simulink subsystem "PvtSubSys_VSM_ALL"  (R2020b)
settings: Solver=VariableStepAuto  StartTime=0.0  StopTime=10.0  RelTol=1e-3
values from neighbouring files (symbols this model uses):
  P_VSM_NOH_Act_Req = 0    [VSM_All.sldd]
  P_VSM_NOH_Swt_Req = 0    [VSM_All.sldd]
undefined symbols (not defined in the file or in its folder): ACC_STATE, HWA_STATE, LCK_STATE, P_VSM_ACCSOS_SW, P_VSM_AESSwtReq, P_VSM_CruiseFunUserInputMappingWays, P_VSM_ELKSwtReq, P_VSM_ESS_VehSwtReq, P_VSM_HWA_DMS_Enable, P_VSM_ICA_HandsOffSwtReq, P_VSM_IntelligentEvaSwtReq, P_VSM_ISLSwtReq, P_VSM_LCKSwtReq, P_VSM_LDWSwtReq, P_VSM_LKASwtReq, P_VSM_LSSSwtReq, P_VSM_PowerTrainConfig, P_VSM_SOSContinueTime, P_VSM_SOSSpdLimit, P_VSM_TSR_Dis_keep_SPL_Table, P_VSM_TSR_Dis_keep_SPLend, P_VSM_TSR_Dis_keep_TS_Table, P_VSM_TSR_Ena_SPLSupp_Table, P_VSM_TSR_Ena_TS_Table, P_VSM_TSR_SLIF_Speed_High, P_VSM_TSR_SLIF_Speed_Low, P_VSM_TSR_SLW_SnvtySwitch, P_VSM_TSR_SLW_Speed_Delta_disable, P_VSM_TSR_SLW_Speed_Delta_enable, P_VSM_TSR_SLW_Speed_High, P_VSM_TSR_SLW_Speed_Low, P_VSM_TSR_SLW_TrafEyeAvtiveDist, P_VSM_TSR_SLW_Warning_Time, P_VSM_TSR_SteerWheelAngle, P_VSM_TSR_SWS_speed_withDir, P_VSM_TSR_SWS_speed_woDir, P_VSM_TSRSwtReq, P_VSM_TSRWarnSwtReq, TJA_STATE, User_LC_ALCswt, User_LC_DrvConfirm, User_LC_DrvLCswt, User_LC_DrvOverride, User_LC_LeTurnNextLineReq, User_LC_RiTurnNextLineReq, User_LC_TurnMostLeLineReq, User_LC_TurnMostRiLineReq, User_LeTurnLmpOn, User_RiTurnLmpOn
libraries: simulink x51
(part 1 of 7)
settings Model: Creator=GW00184765  LastModifiedBy=GW00201118

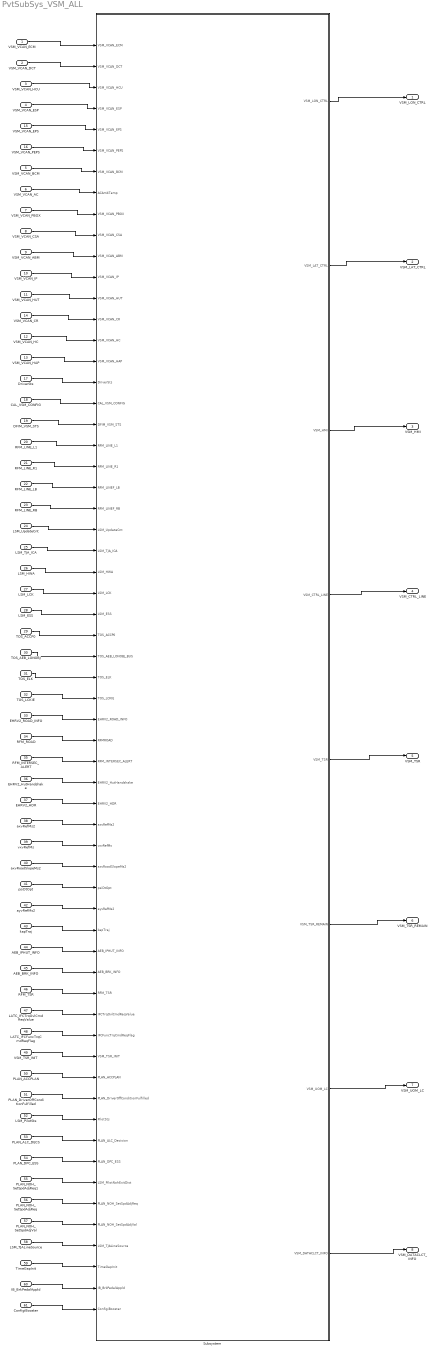
== system PvtSubSys_VSM_ALL ==
  VSM_VCAN_ECM : Inport  OutDataTypeStr=Bus: VCAN_ECM_MSG_BUS  PortDimensions=1  BusOutputAsStruct=on
  VSM_VCAN_DCT : Inport  Port=2  OutDataTypeStr=Bus: VCAN_DCT_MSG_BUS  PortDimensions=1  BusOutputAsStruct=on
  VSM_VCAN_HCU : Inport  Port=3  OutDataTypeStr=Bus: VCAN_HCU_MSG_BUS  PortDimensions=1  BusOutputAsStruct=on
  VSM_VCAN_ESP : Inport  Port=4  OutDataTypeStr=Bus: VCAN_ESP_MSG_BUS  PortDimensions=1  BusOutputAsStruct=on
  VSM_VCAN_BCM : Inport  Port=5  OutDataTypeStr=Bus: VCAN_BCM_MSG_BUS  PortDimensions=1  BusOutputAsStruct=on
  VSM_VCAN_AC : Inport  Port=6  OutDataTypeStr=Bus: VCAN_AC_MSG_BUS  PortDimensions=1  BusOutputAsStruct=on
  VSM_VCAN_PBOX : Inport  Port=7  OutDataTypeStr=Bus: VCAN_PBOX_MSG_BUS  PortDimensions=1  BusOutputAsStruct=on
  VSM_VCAN_CSA : Inport  Port=8  OutDataTypeStr=Bus: VCAN_CSA_MSG_BUS  PortDimensions=1  BusOutputAsStruct=on
  VSM_VCAN_ABM : Inport  Port=9  OutDataTypeStr=Bus: VCAN_ABM_MSG_BUS  PortDimensions=1  BusOutputAsStruct=on
  VSM_VCAN_IP : Inport  Port=10  OutDataTypeStr=Bus: VCAN_IP_MSG_BUS  PortDimensions=1  BusOutputAsStruct=on
  VSM_VCAN_HUT : Inport  Port=11  OutDataTypeStr=Bus: VCAN_HUT_MSG_BUS  PortDimensions=1  BusOutputAsStruct=on
  VSM_VCAN_HC : Inport  Port=12  OutDataTypeStr=Bus: VCAN_HC_MSG_BUS  PortDimensions=1  BusOutputAsStruct=on
  VSM_VCAN_HAP : Inport  Port=13  OutDataTypeStr=Bus: VCAN_HAP_MSG_BUS  PortDimensions=1  BusOutputAsStruct=on
  VSM_VCAN_CR : Inport  Port=14  OutDataTypeStr=Bus: VCAN_CR_MSG_BUS  PortDimensions=1  BusOutputAsStruct=on
  VSM_VCAN_EPS : Inport  Port=15  OutDataTypeStr=Bus: VCAN_EPS_MSG_BUS  PortDimensions=1  BusOutputAsStruct=on
  VSM_VCAN_PEPS : Inport  Port=16  OutDataTypeStr=Bus: VCAN_PEPS_MSG_BUS  PortDimensions=1  BusOutputAsStruct=on
  DriverSts : Inport  Port=17  OutDataTypeStr=uint8  PortDimensions=1  BusOutputAsStruct=on
  CAL_VSM_CONFIG : Inport  Port=18  OutDataTypeStr=Bus: CAL_VSM_CONFIG_BUS  PortDimensions=1  BusOutputAsStruct=on
  DFIM_VSM_STS : Inport  Port=19  OutDataTypeStr=Bus: DFIM_VSM_STS_BUS  PortDimensions=1  BusOutputAsStruct=on
  RFM_LINE_L1 : Inport  Port=20  OutDataTypeStr=Bus: RFM_LINE_BUS  PortDimensions=1  BusOutputAsStruct=on
  RFM_LINE_R1 : Inport  Port=21  OutDataTypeStr=Bus: RFM_LINE_BUS  PortDimensions=1  BusOutputAsStruct=on
  RFM_LINE_LB : Inport  Port=22  OutDataTypeStr=Bus: RFM_LINE_BUS  PortDimensions=1  BusOutputAsStruct=on
  RFM_LINE_RB : Inport  Port=23  OutDataTypeStr=Bus: RFM_LINE_BUS  PortDimensions=1  BusOutputAsStruct=on
  LSM_UpdateCnt : Inport  Port=24  OutDataTypeStr=uint32  PortDimensions=1  BusOutputAsStruct=on
  LSM_TJA_ICA : Inport  Port=25  OutDataTypeStr=Bus: LSM_TJA_ICA_BUS  PortDimensions=1  BusOutputAsStruct=on
  LSM_HWA : Inport  Port=26  OutDataTypeStr=Bus: LSM_HWA_BUS  PortDimensions=1  BusOutputAsStruct=on
  LSM_LCK : Inport  Port=27  OutDataTypeStr=Bus: LSM_LCK_BUS  PortDimensions=1  BusOutputAsStruct=on
  LSM_ESS : Inport  Port=28  OutDataTypeStr=Bus: LSM_ESS_BUS  PortDimensions=1  BusOutputAsStruct=on
  TOS_ACCP0 : Inport  Port=29  OutDataTypeStr=Bus: TOS_ACCP0_BUS  PortDimensions=1  BusOutputAsStruct=on
  TOS_AEB_LONOBJ : Inport  Port=30  OutDataTypeStr=Bus: TOS_AEB_LONOBJ_BUS  PortDimensions=1  BusOutputAsStruct=on
  TOS_ELK : Inport  Port=31  OutDataTypeStr=Bus: TOS_ELK_BUS  PortDimensions=1  BusOutputAsStruct=on
  TOS_LCKIE : Inport  Port=32  OutDataTypeStr=Bus: TOS_LCKIE_BUS  PortDimensions=1  BusOutputAsStruct=on
  EHRV2_ROAD_INFO : Inport  Port=33  OutDataTypeStr=Bus: EHRV2_ROAD_INFO_BUS  PortDimensions=1  BusOutputAsStruct=on
  RFM_ROAD : Inport  Port=34  OutDataTypeStr=Bus: RFM_ROAD_BUS  PortDimensions=1  BusOutputAsStruct=on
  RFM_INTERSEC_ALERT : Inport  Port=35  OutDataTypeStr=Bus: RFM_INTERSEC_ALERT_BUS  PortDimensions=1  BusOutputAsStruct=on
  EHRV2_HutHandshake : Inport  Port=36  OutDataTypeStr=uint8  PortDimensions=1  BusOutputAsStruct=on
  EHRV2_HDR : Inport  Port=37  OutDataTypeStr=Bus: EHRV2_HDR_BUS  PortDimensions=1  BusOutputAsStruct=on
  axvRefMs2 : Inport  Port=38  OutDataTypeStr=single  PortDimensions=1  BusOutputAsStruct=on
  vxvRefMs : Inport  Port=39  OutDataTypeStr=single  PortDimensions=1  BusOutputAsStruct=on
  axvRoadSlopeMs2 : Inport  Port=40  OutDataTypeStr=single  PortDimensions=1  BusOutputAsStruct=on
  psiDtOpt : Inport  Port=41  OutDataTypeStr=single  PortDimensions=1  BusOutputAsStruct=on
  ayvRefMs2 : Inport  Port=42  OutDataTypeStr=single  PortDimensions=1  BusOutputAsStruct=on
  kapTraj : Inport  Port=43  OutDataTypeStr=single  PortDimensions=1  BusOutputAsStruct=on
  AEB_IPHUT_INFO : Inport  Port=44  OutDataTypeStr=Bus: AEB_IPHUT_INFO_BUS  PortDimensions=1  BusOutputAsStruct=on
  AEB_BRK_INFO : Inport  Port=45  OutDataTypeStr=Bus: AEB_BRK_INFO_BUS  PortDimensions=1  BusOutputAsStruct=on
  RFM_TSR : Inport  Port=46  OutDataTypeStr=Bus: RFM_TSR_BUS  PortDimensions=1  BusOutputAsStruct=on
  LATC_IFCTrqOvlCmdReqValue : Inport  Port=47  OutDataTypeStr=single  PortDimensions=1  BusOutputAsStruct=on
  LATC_IFCFuncTrqCmdReqFlag : Inport  Port=48  OutDataTypeStr=uint8  PortDimensions=1  BusOutputAsStruct=on
  VSM_TSR_INIT : Inport  Port=49  OutDataTypeStr=Bus: VSM_TSR_INIT_BUS  PortDimensions=1  BusOutputAsStruct=on
  PLAN_ACCPLAN : Inport  Port=50  OutDataTypeStr=Bus: PLAN_ACCPLAN_BUS  PortDimensions=1  BusOutputAsStruct=on
  PLAN_DriverOffConditionFulfilled : Inport  Port=51  OutDataTypeStr=boolean  PortDimensions=1  BusOutputAsStruct=on
  LSM_PilotSts : Inport  Port=52  OutDataTypeStr=uint8  PortDimensions=1  BusOutputAsStruct=on
  PLAN_ALC_DECS : Inport  Port=53  OutDataTypeStr=Bus: PLAN_ALC_DECS_BUS  PortDimensions=1  BusOutputAsStruct=on
  PLAN_DPC_ESS : Inport  Port=54  OutDataTypeStr=Bus: PLAN_DPC_ESS_BUS  PortDimensions=1  BusOutputAsStruct=on
  PLAN_NOH_SetSpdAdjReq1 : Inport  Port=55  OutDataTypeStr=uint16
  PLAN_NOH_SetSpdAdjReq : Inport  Port=56  OutDataTypeStr=boolean
  PLAN_NOH_SetSpdAdjVal : Inport  Port=57  OutDataTypeStr=uint8
  LSM_TJALineSource : Inport  Port=58  OutDataTypeStr=uint8
  TimeGapInit : Inport  Port=59
  IB_BrkPedalAppld : Inport  Port=60
  ConfigiBooster : Inport  Port=61
  Subsystem : Subsystem
  VSM_LON_CTRL : Outport  OutDataTypeStr=Bus: VSM_LON_CTRL_BUS  PortDimensions=1  BusOutputAsStruct=on
  VSM_LAT_CTRL : Outport  Port=2  OutDataTypeStr=Bus: VSM_LAT_CTRL_BUS  BusOutputAsStruct=on
  VSM_HMI : Outport  Port=3  OutDataTypeStr=Bus: VSM_HMI_BUS  PortDimensions=1  BusOutputAsStruct=on
  VSM_CTRL_LINE : Outport  Port=4  OutDataTypeStr=Bus: VSM_CTRL_LINE_BUS  PortDimensions=1  BusOutputAsStruct=on
  VSM_TSR : Outport  Port=5  OutDataTypeStr=Bus: VSM_TSR_BUS  PortDimensions=1  BusOutputAsStruct=on
  VSM_TSR_REMAIN : Outport  Port=6  OutDataTypeStr=Bus: VSM_TSR_REMAIN_BUS  BusOutputAsStruct=on
  VSM_UOM_LC : Outport  Port=7  OutDataTypeStr=Bus: VSM_UOM_LC_BUS  PortDimensions=1  BusOutputAsStruct=on
  VSM_DATACLCT_INFO : Outport  Port=8  OutDataTypeStr=Bus: VSM_DATACLCT_INFO_BUS  PortDimensions=1  BusOutputAsStruct=on
  wires:
  Subsystem/1(VSM_LON_CTRL) -> VSM_LON_CTRL/1
  Subsystem/2(VSM_LAT_CTRL) -> VSM_LAT_CTRL/1
  Subsystem/3(VSM_HMI) -> VSM_HMI/1
  Subsystem/4(VSM_CTRL_LINE) -> VSM_CTRL_LINE/1
  Subsystem/5(VSM_TSR) -> VSM_TSR/1
  Subsystem/6(VSM_TSR_REMAIN) -> VSM_TSR_REMAIN/1
  Subsystem/7(VSM_UOM_LC) -> VSM_UOM_LC/1
  Subsystem/8(VSM_DATACLCT_INFO) -> VSM_DATACLCT_INFO/1
  VSM_VCAN_ECM/1 -> Subsystem/1(VSM_VCAN_ECM)
  VSM_VCAN_DCT/1 -> Subsystem/2(VSM_VCAN_DCT)
  VSM_VCAN_HCU/1 -> Subsystem/3(VSM_VCAN_HCU)
  VSM_VCAN_ESP/1 -> Subsystem/4(VSM_VCAN_ESP)
  VSM_VCAN_BCM/1 -> Subsystem/7(VSM_VCAN_BCM)
  VSM_VCAN_AC/1 -> Subsystem/8(ACAmbTemp)
  VSM_VCAN_PBOX/1 -> Subsystem/9(VSM_VCAN_PBOX)
  VSM_VCAN_CSA/1 -> Subsystem/10(VSM_VCAN_CSA)
  VSM_VCAN_EPS/1 -> Subsystem/5(VSM_VCAN_EPS)
  VSM_VCAN_PEPS/1 -> Subsystem/6(VSM_VCAN_PEPS)
  VSM_VCAN_ABM/1 -> Subsystem/11(VSM_VCAN_ABM)
  VSM_VCAN_IP/1 -> Subsystem/12(VSM_VCAN_IP)
  VSM_VCAN_HUT/1 -> Subsystem/13(VSM_VCAN_HUT)
  VSM_VCAN_HC/1 -> Subsystem/15(VSM_VCAN_HC)
  VSM_VCAN_HAP/1 -> Subsystem/16(VSM_VCAN_HAP)
  VSM_VCAN_CR/1 -> Subsystem/14(VSM_VCAN_CR)
  DriverSts/1 -> Subsystem/17(DriverSts)
  CAL_VSM_CONFIG/1 -> Subsystem/18(CAL_VSM_CONFIG)
  DFIM_VSM_STS/1 -> Subsystem/19(DFIM_VSM_STS)
  RFM_LINE_L1/1 -> Subsystem/20(RFM_LINE_L1)
  RFM_LINE_R1/1 -> Subsystem/21(RFM_LINE_R1)
  RFM_LINE_LB/1 -> Subsystem/22(RFM_LINEF_LB)
  RFM_LINE_RB/1 -> Subsystem/23(RFM_LINEF_RB)
  LSM_UpdateCnt/1 -> Subsystem/24(LSM_UpdateCnt)
  LSM_TJA_ICA/1 -> Subsystem/25(LSM_TJA_ICA)
  LSM_HWA/1 -> Subsystem/26(LSM_HWA)
  LSM_LCK/1 -> Subsystem/27(LSM_LCK)
  LSM_ESS/1 -> Subsystem/28(LSM_ESS)
  TOS_ACCP0/1 -> Subsystem/29(TOS_ACCP0)
  TOS_AEB_LONOBJ/1 -> Subsystem/30(TOS_AEB_LONOBJ_BUS)
  TOS_ELK/1 -> Subsystem/31(TOS_ELK)
  TOS_LCKIE/1 -> Subsystem/32(TOS_LCKIE)
  EHRV2_ROAD_INFO/1 -> Subsystem/33(EHRV2_ROAD_INFO)
  RFM_ROAD/1 -> Subsystem/34(RFMROAD)
  RFM_INTERSEC_ALERT/1 -> Subsystem/35(RFM_INTERSEC_ALERT)
  EHRV2_HutHandshake/1 -> Subsystem/36(EHRV2_HutHandshake)
  EHRV2_HDR/1 -> Subsystem/37(EHRV2_HDR)
  axvRefMs2/1 -> Subsystem/38(axvRefMs2)
  vxvRefMs/1 -> Subsystem/39(vxvRefMs)
  axvRoadSlopeMs2/1 -> Subsystem/40(axvRoadSlopeMs2)
  psiDtOpt/1 -> Subsystem/41(psiDtOpt)
  ayvRefMs2/1 -> Subsystem/42(ayvRefMs2)
  kapTraj/1 -> Subsystem/43(kapTraj)
  AEB_IPHUT_INFO/1 -> Subsystem/44(AEB_IPHUT_INFO)
  AEB_BRK_INFO/1 -> Subsystem/45(AEB_BRK_INFO)
  RFM_TSR/1 -> Subsystem/46(RFM_TSR)
  LATC_IFCTrqOvlCmdReqValue/1 -> Subsystem/47(IFCTrqOvlCmdReqValue)
  LATC_IFCFuncTrqCmdReqFlag/1 -> Subsystem/48(IFCFuncTrqCmdReqFlag)
  VSM_TSR_INIT/1 -> Subsystem/49(VSM_TSR_INIT)
  PLAN_ACCPLAN/1 -> Subsystem/50(PLAN_ACCPLAN)
  PLAN_DriverOffConditionFulfilled/1 -> Subsystem/51(PLAN_DriverOffConditionFulfilled)
  LSM_PilotSts/1 -> Subsystem/52(PilotSts)
  PLAN_ALC_DECS/1 -> Subsystem/53(PLAN_ALC_Decision)
  PLAN_DPC_ESS/1 -> Subsystem/54(PLAN_DPC_ESS)
  PLAN_NOH_SetSpdAdjReq/1 -> Subsystem/56(PLAN_NOH_SetSpdAdjReq)
  PLAN_NOH_SetSpdAdjVal/1 -> Subsystem/57(PLAN_NOH_SetSpdAdjVal)
  PLAN_NOH_SetSpdAdjReq1/1 -> Subsystem/55(LSM_PilotNohExitDist)
  LSM_TJALineSource/1 -> Subsystem/58(LSM_TJALineSource)
  TimeGapInit/1 -> Subsystem/59(TimeGapInit)
  IB_BrkPedalAppld/1 -> Subsystem/60(IB_BrkPedalAppld)
  ConfigiBooster/1 -> Subsystem/61(ConfigiBooster)

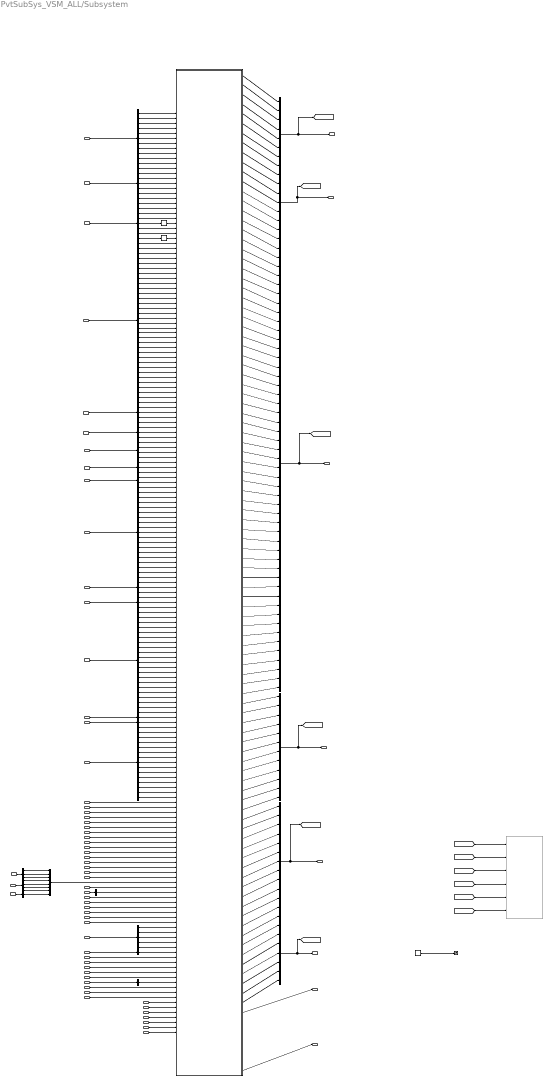
== system PvtSubSys_VSM_ALL/Subsystem ==
  note: 测试版
      | 2021.1.20
      | 1、ACC增加HAP_CAN bus和p0_dx，因此修改框架;
      | 2021.1.22
      | 1、添加LCK居中条件；
      | 2、修改ISL开关逻辑；
      | 2021.1.23
      | UOM添加信号；
      | 2021.1.27
      | TJA_FollowSts修改；
      | 2021.2.1
      | DBC升级4.11
      | 2021.2.22
      | 接口更新NOH；
  VSM_VCAN_ECM : Inport  OutDataTypeStr=Bus: VCAN_ECM_MSG_BUS  BusOutputAsStruct=on
  VSM_VCAN_DCT : Inport  Port=2  OutDataTypeStr=Bus: VCAN_DCT_MSG_BUS  PortDimensions=1  Interpolate=off  BusOutputAsStruct=on
  VSM_VCAN_HCU : Inport  Port=3  OutDataTypeStr=Bus: VCAN_HCU_MSG_BUS  BusOutputAsStruct=on
  VSM_VCAN_ESP : Inport  Port=4  OutDataTypeStr=Bus: VCAN_ESP_MSG_BUS  PortDimensions=1  Interpolate=off  BusOutputAsStruct=on
  VSM_VCAN_EPS : Inport  Port=5  OutDataTypeStr=Bus: VCAN_EPS_MSG_BUS  PortDimensions=1  Interpolate=off  BusOutputAsStruct=on
  VSM_VCAN_PEPS : Inport  Port=6  OutDataTypeStr=Bus: VCAN_PEPS_MSG_BUS  PortDimensions=1  Interpolate=off  BusOutputAsStruct=on
  VSM_VCAN_BCM : Inport  Port=7  OutDataTypeStr=Bus: VCAN_BCM_MSG_BUS  PortDimensions=1  Interpolate=off  BusOutputAsStruct=on
  ACAmbTemp : Inport  Port=8  OutDataTypeStr=Bus: VCAN_AC_MSG_BUS  PortDimensions=1  Interpolate=off  BusOutputAsStruct=on
  VSM_VCAN_PBOX : Inport  Port=9  OutDataTypeStr=Bus: VCAN_PBOX_MSG_BUS  PortDimensions=1  Interpolate=off  BusOutputAsStruct=on
  VSM_VCAN_CSA : Inport  Port=10  OutDataTypeStr=Bus: VCAN_CSA_MSG_BUS  PortDimensions=1  Interpolate=off  BusOutputAsStruct=on
  VSM_VCAN_ABM : Inport  Port=11  OutDataTypeStr=Bus: VCAN_ABM_MSG_BUS  PortDimensions=1  Interpolate=off  BusOutputAsStruct=on
  VSM_VCAN_IP : Inport  Port=12  OutDataTypeStr=Bus: VCAN_IP_MSG_BUS  PortDimensions=1  Interpolate=off  BusOutputAsStruct=on
  VSM_VCAN_HUT : Inport  Port=13  OutDataTypeStr=Bus: VCAN_HUT_MSG_BUS  PortDimensions=1  Interpolate=off  BusOutputAsStruct=on
  VSM_VCAN_CR : Inport  Port=14  OutDataTypeStr=Bus: VCAN_CR_MSG_BUS  PortDimensions=1  Interpolate=off  BusOutputAsStruct=on
  VSM_VCAN_HC : Inport  Port=15  OutDataTypeStr=Bus: VCAN_HC_MSG_BUS  PortDimensions=1  Interpolate=off  BusOutputAsStruct=on
  VSM_VCAN_HAP : Inport  Port=16  OutDataTypeStr=Bus: VCAN_HAP_MSG_BUS  PortDimensions=1  Interpolate=off  BusOutputAsStruct=on
  DriverSts : Inport  Port=17  OutDataTypeStr=uint8  PortDimensions=1  Interpolate=off  BusOutputAsStruct=on
  CAL_VSM_CONFIG : Inport  Port=18  OutDataTypeStr=Bus: CAL_VSM_CONFIG_BUS  PortDimensions=1  Interpolate=off  BusOutputAsStruct=on
  DFIM_VSM_STS : Inport  Port=19  OutDataTypeStr=Bus: DFIM_VSM_STS_BUS  PortDimensions=1  Interpolate=off  BusOutputAsStruct=on
  RFM_LINE_L1 : Inport  Port=20  OutDataTypeStr=Bus: RFM_LINE_BUS  PortDimensions=1  Interpolate=off  BusOutputAsStruct=on
  RFM_LINE_R1 : Inport  Port=21  OutDataTypeStr=Bus: RFM_LINE_BUS  PortDimensions=1  Interpolate=off  BusOutputAsStruct=on
  RFM_LINEF_LB : Inport  Port=22  OutDataTypeStr=Bus: RFM_LINE_BUS  PortDimensions=1  Interpolate=off  BusOutputAsStruct=on
  RFM_LINEF_RB : Inport  Port=23  OutDataTypeStr=Bus: RFM_LINE_BUS  PortDimensions=1  Interpolate=off  BusOutputAsStruct=on
  LSM_UpdateCnt : Inport  Port=24  OutDataTypeStr=uint32  PortDimensions=1  Interpolate=off  BusOutputAsStruct=on
  LSM_TJA_ICA : Inport  Port=25  OutDataTypeStr=Bus: LSM_TJA_ICA_BUS  PortDimensions=1  Interpolate=off  BusOutputAsStruct=on
  LSM_HWA : Inport  Port=26  OutDataTypeStr=Bus: LSM_HWA_BUS  PortDimensions=1  Interpolate=off  BusOutputAsStruct=on
  LSM_LCK : Inport  Port=27  OutDataTypeStr=Bus: LSM_LCK_BUS  PortDimensions=1  Interpolate=off  BusOutputAsStruct=on
  LSM_ESS : Inport  Port=28  OutDataTypeStr=Bus: LSM_ESS_BUS  PortDimensions=1  Interpolate=off  BusOutputAsStruct=on
  TOS_ACCP0 : Inport  Port=29  OutDataTypeStr=Bus: TOS_ACCP0_BUS  PortDimensions=1  BusOutputAsStruct=on
  TOS_AEB_LONOBJ_BUS : Inport  Port=30  OutDataTypeStr=Bus: TOS_AEB_LONOBJ_BUS  PortDimensions=1  BusOutputAsStruct=on
  TOS_ELK : Inport  Port=31  OutDataTypeStr=Bus: TOS_ELK_BUS  PortDimensions=1  BusOutputAsStruct=on
  TOS_LCKIE : Inport  Port=32  OutDataTypeStr=Bus: TOS_LCKIE_BUS  PortDimensions=1  BusOutputAsStruct=on
  EHRV2_ROAD_INFO : Inport  Port=33  OutDataTypeStr=Bus: EHRV2_ROAD_INFO_BUS  PortDimensions=1  Interpolate=off  BusOutputAsStruct=on
  RFMROAD : Inport  Port=34  OutDataTypeStr=Bus: RFM_ROAD_BUS
  RFM_INTERSEC_ALERT : Inport  Port=35  OutDataTypeStr=Bus: RFM_INTERSEC_ALERT_BUS  PortDimensions=1  BusOutputAsStruct=on
  EHRV2_HutHandshake : Inport  Port=36  OutDataTypeStr=uint8  PortDimensions=1  BusOutputAsStruct=on
  EHRV2_HDR : Inport  Port=37  OutDataTypeStr=Bus: EHRV2_HDR_BUS  PortDimensions=1  BusOutputAsStruct=on
  axvRefMs2 : Inport  Port=38  OutDataTypeStr=single  PortDimensions=1  Interpolate=off  BusOutputAsStruct=on
  vxvRefMs : Inport  Port=39  OutDataTypeStr=single  PortDimensions=1  Interpolate=off  BusOutputAsStruct=on
  axvRoadSlopeMs2 : Inport  Port=40  OutDataTypeStr=single  PortDimensions=1  Interpolate=off  BusOutputAsStruct=on
  psiDtOpt : Inport  Port=41  OutDataTypeStr=single  PortDimensions=1  Interpolate=off  BusOutputAsStruct=on
  ayvRefMs2 : Inport  Port=42  OutDataTypeStr=single  PortDimensions=1  Interpolate=off  BusOutputAsStruct=on
  kapTraj : Inport  Port=43  OutDataTypeStr=single  PortDimensions=1  Interpolate=off  BusOutputAsStruct=on
  AEB_IPHUT_INFO : Inport  Port=44  OutDataTypeStr=Bus: AEB_IPHUT_INFO_BUS  PortDimensions=1  Interpolate=off  BusOutputAsStruct=on
  AEB_BRK_INFO : Inport  Port=45  OutDataTypeStr=Bus: AEB_BRK_INFO_BUS  PortDimensions=1  Interpolate=off  BusOutputAsStruct=on
  RFM_TSR : Inport  Port=46  OutDataTypeStr=Bus: RFM_TSR_BUS  PortDimensions=1  Interpolate=off  BusOutputAsStruct=on
  IFCTrqOvlCmdReqValue : Inport  Port=47  OutDataTypeStr=single  PortDimensions=1  Interpolate=off  BusOutputAsStruct=on
  IFCFuncTrqCmdReqFlag : Inport  Port=48  OutDataTypeStr=uint8  PortDimensions=1  Interpolate=off  BusOutputAsStruct=on
  VSM_TSR_INIT : Inport  Port=49  OutDataTypeStr=Bus: VSM_TSR_INIT_BUS  PortDimensions=1  Interpolate=off  BusOutputAsStruct=on
  PLAN_ACCPLAN : Inport  Port=50  OutDataTypeStr=Bus: PLAN_ACCPLAN_BUS  PortDimensions=1  Interpolate=off  BusOutputAsStruct=on
  PLAN_DriverOffConditionFulfilled : Inport  Port=51  OutDataTypeStr=boolean  PortDimensions=1  Interpolate=off  BusOutputAsStruct=on
  PilotSts : Inport  Port=52
  PLAN_ALC_Decision : Inport  Port=53  OutDataTypeStr=Bus: PLAN_ALC_DECS_BUS
  PLAN_DPC_ESS : Inport  Port=54  OutDataTypeStr=Bus: PLAN_DPC_ESS_BUS
  LSM_PilotNohExitDist : Inport  Port=55  OutDataTypeStr=uint16
  PLAN_NOH_SetSpdAdjReq : Inport  Port=56  OutDataTypeStr=boolean
  PLAN_NOH_SetSpdAdjVal : Inport  Port=57  OutDataTypeStr=uint8
  LSM_TJALineSource : Inport  Port=58
  TimeGapInit : Inport  Port=59
  IB_BrkPedalAppld : Inport  Port=60
  ConfigiBooster : Inport  Port=61
  Bus Creator : BusCreator  Inputs=8  OutDataTypeStr=Bus: VSM_LON_CTRL_BUS  NonVirtualBus=on
  Bus Creator1 : BusCreator  Inputs=7  OutDataTypeStr=Bus: VSM_LAT_CTRL_BUS  NonVirtualBus=on
  Bus Creator2 : BusCreator  Inputs=50  OutDataTypeStr=Bus: VSM_HMI_BUS  NonVirtualBus=on
  Bus Creator3 : BusCreator  Inputs=12  OutDataTypeStr=Bus: VSM_CTRL_LINE_BUS  NonVirtualBus=on
  Bus Creator4 : BusCreator  Inputs=13  OutDataTypeStr=Bus: VSM_TSR_BUS  NonVirtualBus=on
  Bus Creator5 : BusCreator  Inputs=7  OutDataTypeStr=Bus: VSM_TSR_REMAIN_BUS  NonVirtualBus=on
  Bus Creator6 : BusCreator  Inputs=8
  Bus Selector : BusSelector  OutputSignals=FrntWshrSwtSts,FrntWiprSwtSts,LTurnLmpSwtSts,RTurnLmpSwtSts,SteerWheelAng,SteerWheelAngSign,SteerWheelSpd,SteerWheelSpdSign,SAS_Sts,ACC_TimeGap_IncSetSwt,ACC_TimeGap_DecSetSwt,CC_ACC_CRUISE_OFFSwt,CC_ACC_CANCEL_OFFSwt,CC_ACC_IncSetSpd_ResuSwt,CC_ACC_DecSetSpd_SetSwt,CC_ACCSwtErr,HWA_OK_OFFSwt
  Bus Selector1 : BusSelector  OutputSignals=HCU_BrkPedalSts,HCU_AccelPedalPosn_Diag,HCU_ACCInterface,HCU_PowertrainSts,ACU_ShiftInProgress,HCU_DrvMod,HCU_PTDrvMod,DrvTrqReqOvld,HCU_GearSts
  Bus Selector10 : BusSelector  OutputSignals=i_func_road_class,i_form_of_way,i_road_curvature_far
  Bus Selector11 : BusSelector  OutputSignals=MapDataValid
  Bus Selector12 : BusSelector  OutputSignals=f_tunnel_distance,b_tunnel,f_bridge_distance,b_bridge
  Bus Selector13 : BusSelector  OutputSignals=f_start_distance
  Bus Selector14 : BusSelector  OutputSignals=EPS_FailSts,EPS_TrqSnsrSts,EPS_SteerMod,EPS_LKATorqOvrlDlvd,EPS_LKATorqOvrlDlvdVld,EPS_LKATrqOvlDlvdSts,EPS_DrvInpTrqVal_HighReslolution
  Bus Selector15 : BusSelector  OutputSignals=SysPowerMod
  Bus Selector16 : BusSelector  OutputSignals=ACAmbTemp
  Bus Selector17 : BusSelector  OutputSignals=IP_VehSpdUnit
  Bus Selector18 : BusSelector  OutputSignals=CR_BrkgReq
  Bus Selector19 : BusSelector  OutputSignals=HighBeamSts_HC
  Bus Selector2 : BusSelector  OutputSignals=CurrentGearValid,SHIFT_IN_PROGRESS,TargetGearValid,TARGET_GEAR,ShiftInPrgValid,CURRENT_GEAR,TGS_LEVER
  Bus Selector26 : BusSelector  OutputSignals=AEB_VehResp,AEB_PedResp,FCW_Warn,AEB_VehTrig,AEB_PedTrig
  Bus Selector27 : BusSelector  OutputSignals=AEB_TgtDecel_Req
  Bus Selector3 : BusSelector  OutputSignals=DrivingModDis,BrkDskOvrheatd,NoBrkForce,VehStandstill,HDCCtrl,CDDActv,CDDAvailable,AVHSts,ESPFuncOffSts,ESPBrkLmpCtrl,ESPFailSts,ESP_MasterCylBrkPressVld,MSRActv,VDCActv,PTCActv,BTCActv,ESP_MasterCylBrkPress,MSRActv_RA,PTCActv_RA,BTCActv_RA,ABSFailSts,EBDFailSts,VehSpd,ABSActv,EPBSts,EPB_SwtPosn,RLWheelDriveDirection,RLWheelSpd,RRWheelDriveDirection,RRWheelSpd
  Bus Selector30 : BusSelector  OutputSignals=EngState_PHEV,EngSpd,EngState,BrkPedalSts,Start_StopSts,AccPedalOverride,AccelPedlPosnDiagc,ECMRespACC,ECMACCInterface,AccelPedalPosn,EngLimpHomeSts
  Bus Selector4 : BusSelector  OutputSignals=ACC_axvCvAim
  Bus Selector5 : BusSelector  OutputSignals=WiprReq_F_PBOX,DrvDoorSts,PassengerDoorSts,WindshldWiprActvSts,HazardLmpSwtSts,KL30BRelaySts
  Bus Selector6 : BusSelector  OutputSignals=HoodSts_F_Pbox,FFogLmpSts_F_Pbox,RFogLmpSts_R_Pbox,LowBeamSts_F_Pbox
  Bus Selector7 : BusSelector  OutputSignals=DrvSBR,PassSBR,VehLgtAccel,VehLatAccel,VehYawRate
  Bus Selector8 : BusSelector  OutputSignals=IFC_SnvtySet,LKASwtReq,LCKSwtReq,ELKSwtReq,ESS_PedSwtReq,ESS_VehSwtReq,LDWSwtReq,TSRSwtReq,TSRWarnSwtReq,ICA_HandsOffSwtReq,ISLSwtReq,TSR_SnvtySet,LSSWarnFormSwtReq,LSSSwtReq,IntelligentEvaSwtReq,AESSwtReq,HWA_SwtReq,HWA_SnvtySet,ALC_SwtReq,NOH_Act_Req,NOH_Swt_Req,NavRoadType
  Bus Selector9 : BusSelector  OutputSignals=USS_FrontSys_Status,USS_FLCNear_Obj_Confidence,USS_FLCNear_Obj_Pos_X,USS_FLCNear_Obj_Pos_Y,USS_FLMNear_Obj_Confidence,USS_FLMNear_Obj_Pos_X,USS_FLMNear_Obj_Pos_Y,USS_FRMNear_Obj_Confidence,USS_FRMNear_Obj_Pos_X,USS_FRMNear_Obj_Pos_Y,USS_FRCNear_Obj_Confidence,USS_FRCNear_Obj_Pos_X,USS_FRCNear_Obj_Pos_Y,APS_WorkSts,DVRWorkSts
  Compare To Constant : simulink/Logic and Bit Operations/Compare To Constant  relop===  const=1  OutDataTypeStr=boolean
  Compare To Constant1 : simulink/Logic and Bit Operations/Compare To Constant  relop===  const=1  OutDataTypeStr=boolean
  Counter Limited : simulink/Sources/Counter Limited  uplimit=15  tsamp=-1
  StateManage : Subsystem
  Terminator1 : Terminator
  VSM_Signal : Subsystem  Commented=on
  VSM_LON_CTRL : Outport  OutDataTypeStr=Bus: VSM_LON_CTRL_BUS  PortDimensions=1  BusOutputAsStruct=on
  VSM_LAT_CTRL : Outport  Port=2  OutDataTypeStr=Bus: VSM_LAT_CTRL_BUS  BusOutputAsStruct=on
  VSM_HMI : Outport  Port=3  OutDataTypeStr=Bus: VSM_HMI_BUS  PortDimensions=1  BusOutputAsStruct=on
  VSM_CTRL_LINE : Outport  Port=4  OutDataTypeStr=Bus: VSM_CTRL_LINE_BUS  PortDimensions=1  BusOutputAsStruct=on
  VSM_TSR : Outport  Port=5  OutDataTypeStr=Bus: VSM_TSR_BUS  PortDimensions=1  BusOutputAsStruct=on
  VSM_TSR_REMAIN : Outport  Port=6  OutDataTypeStr=Bus: VSM_TSR_REMAIN_BUS  BusOutputAsStruct=on
  VSM_UOM_LC : Outport  Port=7  OutDataTypeStr=Bus: VSM_UOM_LC_BUS
  VSM_DATACLCT_INFO : Outport  Port=8  OutDataTypeStr=Bus: VSM_DATACLCT_INFO_BUS  PortDimensions=1  BusOutputAsStruct=on
  wires:
  Bus Selector10/3 -> Bus Creator6/3  "<i_road_curvature_far>"
  ConfigiBooster/1 -> StateManage/185(ConfigiBooster)
  IB_BrkPedalAppld/1 -> StateManage/184(IB_BrkPedalAppld)
  TimeGapInit/1 -> StateManage/183(TimeGapInit)
  StateManage/8(ACC_TimeGapSetHMI) -> Bus Creator/8
  LSM_TJALineSource/1 -> StateManage/182(LSM_TJALineSource)
  StateManage/65(HWA_LaneChange) -> Bus Creator2/50
  StateManage/58(Signal_DriverOffDisp) -> Bus Creator2/43
  StateManage/64(HiPilotModeSelect) -> Bus Creator2/49
  StateManage/63(NOH_DistToExit) -> Bus Creator2/48
  StateManage/62(NOH_SysInfoDisplay) -> Bus Creator2/47
  StateManage/61(NOH_Act_Resp) -> Bus Creator2/46
  StateManage/60(NOH_Swt_Resp) -> Bus Creator2/45
  StateManage/59(NOH_Sts) -> Bus Creator2/44
  LSM_PilotNohExitDist/1 -> StateManage/179(LSM_PilotNohExitDist)
  Bus Selector8/22 -> StateManage/121(NavRoadType)  "<NavRoadType>"
  Bus Selector8/21 -> StateManage/120(NOH_Swt_Req)  "<NOH_Swt_Req>"
  Bus Selector8/20 -> StateManage/119(NOH_Act_Req)  "<NOH_Act_Req>"
  StateManage/104(VSM_DATACLCT_INFO) -> VSM_DATACLCT_INFO/1
  Compare To Constant1/1 -> StateManage/26(DrvTrqReqOvld)
  Compare To Constant/1 -> StateManage/23(ACU_ShiftInProgress)
  Bus Selector19/1 -> StateManage/123(HighBeamSts)  "<HighBeamSts_HC>"
  VSM_VCAN_CR/1 -> Bus Selector18/1
  VSM_VCAN_IP/1 -> Bus Selector17/1
  ACAmbTemp/1 -> Bus Selector16/1
  VSM_VCAN_PEPS/1 -> Bus Selector15/1
  VSM_VCAN_EPS/1 -> Bus Selector14/1
  PLAN_NOH_SetSpdAdjVal/1 -> StateManage/181(PLAN_NOH_SetSpdAdjVal)
  PLAN_NOH_SetSpdAdjReq/1 -> StateManage/180(PLAN_NOH_SetSpdAdjReq)
  StateManage/98(VSM_UOM_LC) -> VSM_UOM_LC/1
  StateManage/57(HWA_TurnLightReq) -> Bus Creator2/42
  Bus Selector13/1 -> Bus Creator6/8  "<f_start_distance>"
  Bus Selector12/4 -> Bus Creator6/7  "<b_bridge>"
  Bus Selector12/3 -> Bus Creator6/6  "<f_bridge_distance>"
  Bus Selector12/2 -> Bus Creator6/5  "<b_tunnel>"
  Bus Selector12/1 -> Bus Creator6/4  "<f_tunnel_distance>"
  Bus Selector10/2 -> Bus Creator6/2  "<i_form_of_way>"
  Bus Selector10/1 -> Bus Creator6/1  "<i_func_road_class>"
  RFM_INTERSEC_ALERT/1 -> Bus Selector13/1
  RFMROAD/1 -> Bus Selector12/1
  EHRV2_ROAD_INFO/1 -> Bus Selector10/1
  EHRV2_HDR/1 -> Bus Selector11/1
  LSM_TJA_ICA/1 -> StateManage/147(LSM_TJA_ICA)
  [VSM_HMI] -> VSM_Signal/3(VSM_HMI)  "VSM_HMI"
  Bus Selector3/28 -> StateManage/55(RLWheelSpd)  "<RLWheelSpd>"
  Bus Selector18/1 -> StateManage/122(CR_BrkgReq)  "<CR_BrkgReq>"
  Bus Selector30/10 -> StateManage/10(AccelPedalPosn)  "<AccelPedalPosn>"
  StateManage/4(ACC_TimeGapSet) -> Bus Creator/4
  axvRefMs2/1 -> StateManage/158(axvRefMs2)
  StateManage/93(TS_SignName_Dist_Remain) -> Bus Creator5/3
  Bus Selector1/6 -> StateManage/24(HCU_DrvMod)  "<HCU_DrvMod>"
  Bus Selector15/1 -> StateManage/65(SysPowerMod)  "<SysPowerMod>"
  Bus Selector9/10 -> StateManage/133(USS_FRMNear_Obj_Pos_Y)  "<USS_FRMNear_Obj_Pos_Y>"
  Bus Selector1/7 -> StateManage/25(HCU_PTDrvMod)  "<HCU_PTDrvMod>"
  StateManage/42(HWA_SnvtySet_Resp) -> Bus Creator2/27
  StateManage/96(TS_SignName_Value_Remain) -> Bus Creator5/6
  StateManage/92(SPL_whSupp_Dist_Remain) -> Bus Creator5/2
  StateManage/88(TSRConSpdLimWarn) -> Bus Creator4/11
  StateManage/79(TSRResp) -> Bus Creator4/2
  StateManage/82(TSRSpdLimUnit) -> Bus Creator4/5
  VSM_VCAN_ABM/1 -> Bus Selector7/1
  Bus Selector5/5 -> StateManage/70(HazardLmpSwtSts)  "<HazardLmpSwtSts>"
  VSM_VCAN_HCU/1 -> Bus Selector1/1
  Bus Selector5/4 -> StateManage/69(WindshldWiprActvSts)  "<WindshldWiprActvSts>"
  StateManage/3(SetSpeedKmh) -> Bus Creator/3
  Bus Selector3/27 -> StateManage/54(RLWheelDriveDirection)  "<RLWheelDriveDirection>"
  axvRoadSlopeMs2/1 -> StateManage/160(axvRoadSlopeMs2)
  Bus Selector26/3 -> StateManage/166(Inter_FCW_Warn)  "<FCW_Warn>"
  StateManage/81(TSR_Snvty) -> Bus Creator4/4
  StateManage/84(TSRSpdLim) -> Bus Creator4/7
  TOS_ACCP0/1 -> StateManage/151(TOS_ACCP0)
  StateManage/83(TSRSpdLimSts) -> Bus Creator4/6
  StateManage/76(ELKLineC0) -> Bus Creator3/11
  Bus Creator/1 -> [VSM_LON_CTRL], VSM_LON_CTRL/1
  StateManage/44(ICA_HandsOffSwtResp) -> Bus Creator2/29
  vxvRefMs/1 -> StateManage/159(vxvRefMs)
  StateManage/30(LCKSts) -> Bus Creator2/15
  Bus Selector14/5 -> StateManage/62(EPS_LKATorqOvrlDlvdVld)  "<EPS_LKATorqOvrlDlvdVld>"
  Bus Selector/14 -> StateManage/90(CC_ACC_IncSetSpd_ResuSwt)  "<CC_ACC_IncSetSpd_ResuSwt>"
  StateManage/75(ELKLineC1) -> Bus Creator3/10
  StateManage/40(EPBTakeOver_Req) -> Bus Creator2/25
  PLAN_DriverOffConditionFulfilled/1 -> StateManage/170(DriveOffConditionFulfilled)
  VSM_VCAN_ESP/1 -> Bus Selector3/1
  Bus Selector7/3 -> StateManage/96(VehLgtAccel)  "<VehLgtAccel>"
  StateManage/50(DriverInloop_Monitor) -> Bus Creator2/35
  StateManage/67(LKALineC3) -> Bus Creator3/2
  PLAN_ALC_Decision/1 -> StateManage/176(ALC)
  Bus Selector3/24 -> StateManage/51(ABSActv)  "<ABSActv>"
  Bus Selector/16 -> StateManage/92(CC_ACCSwtErr)  "<CC_ACCSwtErr>"
  Bus Selector8/7 -> StateManage/106(LDWSwtReq)  "<LDWSwtReq>"
  StateManage/54(ESSSts) -> Bus Creator2/39
  VSM_VCAN_BCM/1 -> Bus Selector5/1
  kapTraj/1 -> StateManage/163(kapTraj)
  StateManage/70(LKALineC0) -> Bus Creator3/5
  StateManage/38(ISL_InterSysInfoDisp) -> Bus Creator2/23
  Bus Selector8/1 -> StateManage/100(IFC_SnvtySet)  "<IFC_SnvtySet>"
  StateManage/73(ELKLineC3) -> Bus Creator3/8
  Bus Selector3/8 -> StateManage/35(AVHSts)  "<AVHSts>"
  TOS_LCKIE/1 -> StateManage/154(TOS_LCKIE)
  StateManage/1(ACCSts) -> Bus Creator/1
  StateManage/53(TJA_FollowSts) -> Bus Creator2/38
  VSM_VCAN_DCT/1 -> Bus Selector2/1
  StateManage/31(HandsOffWarningLevel) -> Bus Creator2/16
  Bus Selector9/9 -> StateManage/132(USS_FRMNear_Obj_Pos_X)  "<USS_FRMNear_Obj_Pos_X>"
  Bus Selector3/15 -> StateManage/42(PTCActv)  "<PTCActv>"
  StateManage/78(TSRSts) -> Bus Creator4/1
  RFM_LINE_R1/1 -> StateManage/143(RFM_LINE_R1)
  StateManage/55(AESSts) -> Bus Creator2/40
  RFM_TSR/1 -> StateManage/171(RFM_TSR)
  Bus Selector30/1 -> StateManage/1(EngState_PHEV)  "<EngState_PHEV>"
  Bus Selector8/16 -> StateManage/115(AESSwtReq)  "<AESSwtReq>"
  StateManage/69(LKALineC1) -> Bus Creator3/4
  Bus Selector14/4 -> StateManage/61(EPS_LKATorqOvrlDlvd)  "<EPS_LKATorqOvrlDlvd>"
  VSM_VCAN_HAP/1 -> Bus Selector9/1
  StateManage/33(LKASts) -> Bus Creator2/18
  StateManage/52(LaneAvailability) -> Bus Creator2/37
  Bus Selector9/3 -> StateManage/126(USS_FLCNear_Obj_Pos_X)  "<USS_FLCNear_Obj_Pos_X>"
  Bus Selector/12 -> StateManage/88(CC_ACC_CRUISE_OFFSwt)  "<CC_ACC_CRUISE_OFFSwt>"
  StateManage/77(ELKLineRange) -> Bus Creator3/12
  Bus Selector1/3 -> StateManage/21(HCU_ACCInterface)  "<HCU_ACCInterface>"
  LSM_LCK/1 -> StateManage/149(LSM_LCK)
  Bus Selector2/7 -> StateManage/18(TGS_LEVER)  "<TGS_LEVER>"
  Bus Selector2/5 -> StateManage/16(ShiftInPrgValid)  "<ShiftInPrgValid>"
  Bus Selector1/4 -> StateManage/22(HCU_PowertrainSts)  "<HCU_PowertrainSts>"
  Bus Selector1/9 -> StateManage/27(HCU_GearSts)  "<HCU_GearSts>"
  Bus Selector3/14 -> StateManage/41(VDCActv)  "<VDCActv>"
  Bus Selector3/4 -> StateManage/31(VehStandstill)  "<VehStandstill>"
  Bus Selector2/3 -> StateManage/14(TargetGearValid)  "<TargetGearValid>"
  Bus Selector3/26 -> StateManage/53(EPB_SwtPosn)  "<EPB_SwtPosn>"
  StateManage/35(ELKSts) -> Bus Creator2/20
  Bus Selector/17 -> StateManage/93(HWA_OK_OFFSwt)  "<HWA_OK_OFFSwt>"
  StateManage/71(LKALineRange) -> Bus Creator3/6
  Bus Selector8/9 -> StateManage/108(TSRWarnSwtReq)  "<TSRWarnSwtReq>"
  Bus Selector30/8 -> StateManage/8(ECMRespACC)  "<ECMRespACC>"
  TOS_ELK/1 -> StateManage/153(TOS_ELK)
  StateManage/87(TSRConSpdLim) -> Bus Creator4/10
  Bus Selector3/16 -> StateManage/43(BTCActv)  "<BTCActv>"
  Bus Selector8/15 -> StateManage/114(IntelligentEvaSwtReq)  "<IntelligentEvaSwtReq>"
  Bus Selector/6 -> StateManage/82(SteerWheelAngSign)  "<SteerWheelAngSign>"
  CAL_VSM_CONFIG/1 -> StateManage/140(CAL_VSM_CONFIG)
  Bus Selector8/13 -> StateManage/112(LSSWarnFormSwtReq)  "<LSSWarnFormSwtReq>"
  Bus Selector3/12 -> StateManage/39(ESP_MasterCylBrkPressVld)  "<ESP_MasterCylBrkPressVld>"
  Bus Selector/15 -> StateManage/91(CC_ACC_DecSetSpd_SetSwt)  "<CC_ACC_DecSetSpd_SetSwt>"
  Bus Selector8/19 -> StateManage/118(ALC_SwtReq)  "<ALC_SwtReq>"
  Bus Selector9/6 -> StateManage/129(USS_FLMNear_Obj_Pos_X)  "<USS_FLMNear_Obj_Pos_X>"
  Bus Selector/7 -> StateManage/83(SteerWheelSpd)  "<SteerWheelSpd>"
  VSM_VCAN_ECM/1 -> Bus Selector30/1
  Bus Selector2/4 -> StateManage/15(TARGET_GEAR)  "<TARGET_GEAR>"
  StateManage/16(TJASts) -> Bus Creator2/1
  Bus Selector26/5 -> StateManage/168(AEB_PedTrig)  "<AEB_PedTrig>"
  StateManage/18(HWAActive) -> Bus Creator2/3
  Bus Selector2/6 -> StateManage/17(CURRENT_GEAR)  "<CURRENT_GEAR>"
  StateManage/28(CCTextDisp) -> Bus Creator2/13
  AEB_IPHUT_INFO/1 -> Bus Selector26/1
  StateManage/2(ACC_SpdSetValue) -> Bus Creator/2
  Bus Selector8/2 -> StateManage/101(LKASwtReq)  "<LKASwtReq>"
  StateManage/27(TJATextDisp) -> Bus Creator2/12
  StateManage/29(HWATextDisp) -> Bus Creator2/14
  StateManage/36(LCKIEDist) -> Bus Creator2/21
  Bus Selector9/15 -> StateManage/138(DVRWorkSts)  "<DVRWorkSts>"
  Bus Selector/9 -> StateManage/85(SAS_Sts)  "<SAS_Sts>"
  AEB_BRK_INFO/1 -> Bus Selector27/1
  Bus Selector27/1 -> StateManage/169(" ")  "<AEB_TgtDecel_Req>"
  Bus Selector8/4 -> StateManage/103(ELKSwtReq)  "<ELKSwtReq>"
  Bus Selector/3 -> StateManage/79(LTurnLmpSwtSts)  "<LTurnLmpSwtSts>"
  Bus Selector/2 -> StateManage/78(FrntWiprSwtSts)  "<FrntWiprSwtSts>"
  StateManage/23(HWA_ModeDisp) -> Bus Creator2/8
  IFCTrqOvlCmdReqValue/1 -> StateManage/172(epsTrqReqValue)
  [VSM_LAT_CTRL] -> VSM_Signal/2(VSM_LAT_CTRL)  "VSM_LAT_CTRL"
  RFM_LINEF_RB/1 -> StateManage/145(RFM_LINEF_RB)
  StateManage/91(SPL_noSupp_Dist_Remain) -> Bus Creator5/1
  PLAN_DPC_ESS/1 -> StateManage/177(PLAN_DPC_ESS)
  Bus Selector6/1 -> StateManage/73(HoodSts_F_Pbox)  "<HoodSts_F_Pbox>"
  Bus Selector3/13 -> StateManage/40(MSRActv)  "<MSRActv>"
  StateManage/20(ACC_ModeDisp) -> Bus Creator2/5
  VSM_VCAN_HC/1 -> Bus Selector19/1
  Bus Selector14/6 -> StateManage/63(EPS_LKATrqOvlDlvdSts)  "<EPS_LKATrqOvlDlvdSts>"
  Bus Creator1/1 -> [VSM_LAT_CTRL], VSM_LAT_CTRL/1
  Bus Selector14/2 -> StateManage/59(EPS_TrqSnsrSts)  "<EPS_TrqSnsrSts>"
  Bus Creator4/1 -> VSM_TSR/1, [VSM_TSR]
  Bus Selector3/21 -> StateManage/48(ABSFailSts)  "<ABSFailSts>"
  Bus Selector/5 -> StateManage/81(SteerWheelAng)  "<SteerWheelAng>"
  StateManage/95(SPL_whSupp_Value_Remain) -> Bus Creator5/5
  Bus Selector9/12 -> StateManage/135(USS_FRCNear_Obj_Pos_X)  "<USS_FRCNear_Obj_Pos_X>"
  Bus Selector30/9 -> StateManage/9(ECMACCInterface)  "<ECMACCInterface>"
  Bus Selector30/3 -> StateManage/3(EngState)  "<EngState>"
  StateManage/80(TSRWarnResp) -> Bus Creator4/3
  Bus Selector8/12 -> StateManage/111(TSR_SnvtySet)  "<TSR_SnvtySet>"
  Bus Selector3/20 -> StateManage/47(BTCActv_RA)  "<BTCActv_RA>"
  Bus Selector9/1 -> StateManage/124(USS_FrontSys_Status)  "<USS_FrontSys_Status>"
  StateManage/94(SPL_noSupp_Value_Remain) -> Bus Creator5/4
  Bus Creator5/1 -> VSM_TSR_REMAIN/1, [VSM_TSR_REMAIN]
  Bus Selector11/1 -> StateManage/157(MapDataValid)  "<MapDataValid>"
  Bus Selector3/10 -> StateManage/37(ESPBrkLmpCtrl)  "<ESPBrkLmpCtrl>"
  RFM_LINEF_LB/1 -> StateManage/144(RFM_LINEF_LB)
  StateManage/86(TSRSpdLimWarn) -> Bus Creator4/9
  StateManage/72(ELKLineValid) -> Bus Creator3/7
  Bus Selector14/7 -> StateManage/64(EPS_DrvInpTrqVal_HighReslolution)  "<EPS_DrvInpTrqVal_HighReslolution>"
  LSM_UpdateCnt/1 -> StateManage/146(LSM_Cnt)
  Bus Selector8/11 -> StateManage/110(ISLSwtReq)  "<ISLSwtReq>"
  Bus Selector8/8 -> StateManage/107(TSRSwtReq)  "<TSRSwtReq>"
  Bus Creator6/1 -> StateManage/155(EHRV2_ALL)
  StateManage/66(LKALineValid) -> Bus Creator3/1
  StateManage/90(TSRTrfcSignValCfdc) -> Bus Creator4/13
  Bus Selector17/1 -> StateManage/99(IP_VehSpdUnit)  "<IP_VehSpdUnit>"
  Bus Selector30/11 -> StateManage/11(EngLimpHomeSts)  "<EngLimpHomeSts>"
  Bus Selector3/17 -> StateManage/44(ESP_MasterCylBrkPress)  "<ESP_MasterCylBrkPress>"
  StateManage/17(HWASts) -> Bus Creator2/2
  StateManage/32(LDWSts) -> Bus Creator2/17
  Bus Selector3/2 -> StateManage/29(BrkDskOvrheatd)  "<BrkDskOvrheatd>"
  Bus Selector3/11 -> StateManage/38(ESPFailSts)  "<ESPFailSts>"
  Bus Selector9/11 -> StateManage/134(USS_FRCNear_Obj_Confidence)  "<USS_FRCNear_Obj_Confidence>"
  Bus Selector9/2 -> StateManage/125(USS_FLCNear_Obj_Confidence)  "<USS_FLCNear_Obj_Confidence>"
  Bus Selector8/18 -> StateManage/117(HWA_SnvtySet)  "<HWA_SnvtySet>"
  StateManage/12(TarLineC1) -> Bus Creator1/4
  Bus Selector6/2 -> StateManage/74(FFogLmpSts_F_Pbox)  "<FFogLmpSts_F_Pbox>"
  TOS_AEB_LONOBJ_BUS/1 -> StateManage/152(TOS_AEB_LONOBJ_BUS)
  Bus Selector26/1 -> StateManage/164(AEB_VehResp)  "<AEB_VehResp>"
  Bus Selector9/5 -> StateManage/128(USS_FLMNear_Obj_Confidence)  "<USS_FLMNear_Obj_Confidence>"
  VSM_VCAN_PBOX/1 -> Bus Selector6/1
  StateManage/11(TarLineC2) -> Bus Creator1/3
  Bus Selector7/5 -> StateManage/98(VehYawRate)  "<VehYawRate>"
  StateManage/46(HWA_LaneChangeReq) -> Bus Creator2/31
  Bus Selector3/23 -> StateManage/50(VehSpd)  "<VehSpd>"
  StateManage/6(HWAAccControlSts) -> Bus Creator/6
  StateManage/9(TarLineValid) -> Bus Creator1/1
  Bus Selector26/4 -> StateManage/167(AEB_VehTrig)  "<AEB_VehTrig>"
  StateManage/34(LKAWarning) -> Bus Creator2/19
  StateManage/74(ELKLineC2) -> Bus Creator3/9
  Bus Selector5/6 -> StateManage/71("KL30BRelaySts ")  "<KL30BRelaySts>"
  Bus Selector5/3 -> StateManage/68(PassengerDoorSts)  "<PassengerDoorSts>"
  EHRV2_HutHandshake/1 -> StateManage/156(IFCHUTInterface)
  Bus Selector14/1 -> StateManage/58(EPS_FailSts)  "<EPS_FailSts>"
  Bus Selector30/2 -> StateManage/2(EngSpd)  "<EngSpd>"
  [VSM_TSR] -> VSM_Signal/5(VSM_TSR)  "VSM_TSR"
  StateManage/97(SPL_SuppName_Value_Remain) -> Bus Creator5/7
  Bus Selector3/6 -> StateManage/33(CDDActv)  "<CDDActv>"
  Bus Selector6/4 -> StateManage/76(LowBeamSts)  "<LowBeamSts_F_Pbox>"
  StateManage/26(ACCTextDisp) -> Bus Creator2/11
  LSM_ESS/1 -> StateManage/150(LSM_ESS)
  PLAN_ACCPLAN/1 -> Bus Selector4/1
  StateManage/24(HWASlowRetreat_b) -> Bus Creator2/9
  StateManage/21(ACC_ParkShiftReq) -> Bus Creator2/6
  StateManage/43(HWA_Resp) -> Bus Creator2/28
  Bus Selector/10 -> StateManage/86(ACC_TimeGap_IncSetSwt)  "<ACC_TimeGap_IncSetSwt>"
  psiDtOpt/1 -> StateManage/161(psiDtOpt)
  StateManage/49(LSS_WarnFormSwtResp) -> Bus Creator2/34
  Bus Selector/11 -> StateManage/87(ACC_TimeGap_DecSetSwt)  "<ACC_TimeGap_DecSetSwt>"
  Bus Selector3/22 -> StateManage/49(EBDFailSts)  "<EBDFailSts>"
  Bus Selector16/1 -> StateManage/72(ACAmbTemp)  "<ACAmbTemp>"
  Bus Selector3/3 -> StateManage/30(NoBrkForce)  "<NoBrkForce>"
  StateManage/41(ALC_Resp) -> Bus Creator2/26
  PilotSts/1 -> StateManage/178(PilotSts)
  Bus Selector8/3 -> StateManage/102(LCKSwtReq)  "<LCKSwtReq>"
  [VSM_LON_CTRL] -> VSM_Signal/1(VSM_LON_CTRL)  "VSM_LON_CTRL"
  Bus Selector3/30 -> StateManage/57(RRWheelSpd)  "<RRWheelSpd>"
  Bus Selector8/10 -> StateManage/109(ICA_HandsOffSwtReq)  "<ICA_HandsOffSwtReq>"
  Bus Selector9/13 -> StateManage/136(USS_FRCNear_Obj_Pos_Y)  "<USS_FRCNear_Obj_Pos_Y>"
  VSM_VCAN_CSA/1 -> Bus Selector/1
  VSM_TSR_INIT/1 -> StateManage/174(VSM_TSR_INIT)
  IFCFuncTrqCmdReqFlag/1 -> StateManage/173(epsTrqReqFlag)
  StateManage/51(ACC_SOS_Req) -> Bus Creator2/36
  StateManage/39(ISLActive) -> Bus Creator2/24
  [VSM_TSR_REMAIN] -> VSM_Signal/6(VSM_TSR_REMAIN)  "VSM_TSR_REMAIN"
  StateManage/7(ACC_DrvOffReq) -> Bus Creator/7
  Bus Selector8/17 -> StateManage/116(HWA_SwtReq)  "<HWA_SwtReq>"
  Bus Selector7/1 -> StateManage/94(DrvSBR)  "<DrvSBR>"
  StateManage/19(ACC_HazActv) -> Bus Creator2/4
  Bus Selector30/4 -> StateManage/4(BrkPedalSts)  "<BrkPedalSts>"
  StateManage/89(TSRTrfcSignVal) -> Bus Creator4/12
  StateManage/47(HWA_Warning) -> Bus Creator2/32
  Bus Selector7/2 -> StateManage/95(PassSBR)  "<PassSBR>"
  Bus Selector/8 -> StateManage/84(SteerWheelSpdSign)  "<SteerWheelSpdSign>"
  StateManage/37(ACC_ISLResp) -> Bus Creator2/22
  StateManage/25(CruiseChauffeur_ModeDisp) -> Bus Creator2/10
  Bus Selector14/3 -> StateManage/60(EPS_SteerMod)  "<EPS_SteerMod>"
  Bus Selector9/8 -> StateManage/131(USS_FRMNear_Obj_Confidence)  "<USS_FRMNear_Obj_Confidence>"
  StateManage/13(TarLineC0) -> Bus Creator1/5
  Bus Selector2/2 -> StateManage/13(SHIFT_IN_PROGRESS)  "<SHIFT_IN_PROGRESS>"
  Bus Selector9/4 -> StateManage/127(USS_FLCNear_Obj_Pos_Y)  "<USS_FLCNear_Obj_Pos_Y>"
  StateManage/56(LCKIESts) -> Bus Creator2/41
  StateManage/68(LKALineC2) -> Bus Creator3/3
  Bus Selector3/9 -> StateManage/36(ESPFuncOffSts)  "<ESPFuncOffSts>"
  VSM_VCAN_HUT/1 -> Bus Selector8/1
  StateManage/5(vSetBelowMin) -> Bus Creator/5
  Bus Selector1/1 -> StateManage/19(HCU_BrkPedalSts)  "<HCU_BrkPedalSts>"
  Bus Selector8/14 -> StateManage/113(LSSSwtReq)  "<LSSSwtReq>"
  StateManage/10(TarLineC3) -> Bus Creator1/2
  LSM_HWA/1 -> StateManage/148(LSM_HWA)
  Bus Selector5/2 -> StateManage/67(DrvDoorSts)  "<DrvDoorSts>"
  DriverSts/1 -> StateManage/139(DriverSts)
  Bus Selector26/2 -> StateManage/165(AEB_PedResp)  "<AEB_PedResp>"
  Counter Limited/1 -> Terminator1/1  "VSM_Counter"
  Bus Selector3/18 -> StateManage/45(MSRActv_RA)  "<MSRActv_RA>"
  Bus Selector9/7 -> StateManage/130(USS_FLMNear_Obj_Pos_Y)  "<USS_FLMNear_Obj_Pos_Y>"
  Bus Selector2/1 -> StateManage/12(CurrentGearValid)  "<CurrentGearValid>"
  Bus Selector3/5 -> StateManage/32(HDCCtrl)  "<HDCCtrl>"
  ayvRefMs2/1 -> StateManage/162(ayvRefMs2)
  Bus Selector5/1 -> StateManage/66(WiprReq)  "<WiprReq_F_PBOX>"
  RFM_LINE_L1/1 -> StateManage/142(RFM_LINE_L1)
  Bus Selector/4 -> StateManage/80(RTurnLmpSwtSts)  "<RTurnLmpSwtSts>"
  Bus Creator2/1 -> VSM_HMI/1, [VSM_HMI]
  StateManage/85(TSRSpdLimCfdc) -> Bus Creator4/8
  Bus Selector30/7 -> StateManage/7(AccelPedlPosnDiagc)  "<AccelPedlPosnDiagc>"
  DFIM_VSM_STS/1 -> StateManage/141(DFIM_VSM_STS)
  Bus Selector8/6 -> StateManage/105(ESS_VehSwtReq)  "<ESS_VehSwtReq>"
  Bus Creator3/1 -> [VSM_CTRL_LINE], VSM_CTRL_LINE/1
  Bus Selector8/5 -> StateManage/104(ESS_PedSwtReq)  "<ESS_PedSwtReq>"
  Bus Selector30/6 -> StateManage/6(AccPedalOverride)  "<AccPedalOverride>"
  Bus Selector7/4 -> StateManage/97(VehLatAccel)  "<VehLatAccel>"
  Bus Selector30/5 -> StateManage/5(Start_StopSts)  "<Start_StopSts>"
  Bus Selector3/29 -> StateManage/56(RRWheelDriveDirection)  "<RRWheelDriveDirection>"
  Bus Selector1/2 -> StateManage/20(HCU_AccelPedalPosn_Diag)  "<HCU_AccelPedalPosn_Diag>"
  StateManage/45(TJA_ACC_SelSts) -> Bus Creator2/30
  Bus Selector1/5 -> Compare To Constant/1  "<ACU_ShiftInProgress>"
  Bus Selector3/1 -> StateManage/28(DrivingModDis)  "<DrivingModDis>"
  Bus Selector3/25 -> StateManage/52(EPBSts)  "<EPBSts>"
  StateManage/15(TarDangerLevel) -> Bus Creator1/7
  Bus Selector3/19 -> StateManage/46(PTCActv_RA)  "<PTCActv_RA>"
  Bus Selector/1 -> StateManage/77(FrntWshrSwtSts)  "<FrntWshrSwtSts>"
  StateManage/22(TJA_ModeDisp) -> Bus Creator2/7
  [VSM_CTRL_LINE] -> VSM_Signal/4(VSM_CTRL_LINE)  "VSM_CTRL_LINE"
  StateManage/14(TarLineRange) -> Bus Creator1/6
  Bus Selector4/1 -> StateManage/175(Longctrl_Decel_ReqValue)  "<ACC_axvCvAim>"
  StateManage/48(HandsOffDetd) -> Bus Creator2/33
  Bus Selector6/3 -> StateManage/75(RFogLmpSts_R_Pbox)  "<RFogLmpSts_R_Pbox>"
  Bus Selector3/7 -> StateManage/34(CDDAvailable)  "<CDDAvailable>"
  Bus Selector1/8 -> Compare To Constant1/1  "<DrvTrqReqOvld>"
  Bus Selector9/14 -> StateManage/137(APS_WorkSts)  "<APS_WorkSts>"
  Bus Selector/13 -> StateManage/89(CC_ACC_CANCEL_OFFSwt)  "<CC_ACC_CANCEL_OFFSwt>"
